simulink model "fft_wideband_real"  (R2012b)
settings: Solver=ode45  StartTime=0.0  StopTime=19999  RelTol=1e-3
undefined symbols (not defined in the file): fft_wideband_real_shift_schedule_user_data_out
libraries: xbsIndex_r4 x8703, xbsReplacements_r4 x36, xps_library x24, dspsigops x16, simulink_xsg_bridge x1
(part 5 of 51)

== system fft_wideband_real/fft_wideband_real/fft_direct/butterfly2_4 ==
  a : Inport
  b : Inport  Port=2
  w : Inport  Port=3
  sync : Inport  Port=4
  shift : Inport  Port=5
  AddSub0 : xbsIndex_r4/AddSub  mode=Addition  use_carryin=off  use_carryout=off  en=off  latency=2  precision=Full  arith_type=Unsigned  n_bits=16  bin_pt=14  quantization=Truncate  overflow=Wrap  dbl_ovrd=off  use_behavioral_HDL=on  hw_selection=Fabric  pipelined=off  block_type=addsub
  AddSub1 : xbsIndex_r4/AddSub  mode=Addition  use_carryin=off  use_carryout=off  en=off  latency=2  precision=Full  arith_type=Unsigned  n_bits=16  bin_pt=14  quantization=Truncate  overflow=Wrap  dbl_ovrd=off  use_behavioral_HDL=on  hw_selection=Fabric  pipelined=off  block_type=addsub
  AddSub2 : xbsIndex_r4/AddSub  mode=Subtraction  use_carryin=off  use_carryout=off  en=off  latency=2  precision=Full  arith_type=Unsigned  n_bits=16  bin_pt=14  quantization=Truncate  overflow=Wrap  dbl_ovrd=off  use_behavioral_HDL=on  hw_selection=Fabric  pipelined=off  block_type=addsub
  AddSub3 : xbsIndex_r4/AddSub  mode=Subtraction  use_carryin=off  use_carryout=off  en=off  latency=2  precision=Full  arith_type=Unsigned  n_bits=16  bin_pt=14  quantization=Truncate  overflow=Wrap  dbl_ovrd=off  use_behavioral_HDL=on  hw_selection=Fabric  pipelined=off  block_type=addsub
  Logical : xbsIndex_r4/Logical  logical_function=OR  inputs=4  en=off  latency=0  precision=Full  arith_type=Unsigned  n_bits=16  bin_pt=0  align_bp=on  dbl_ovrd=off  block_type=logical
  conv_of_1 : Subsystem
      settings: AttributesFormatString=[20,18]->[18,17]
  conv_of_2 : Subsystem
      settings: AttributesFormatString=[20,18]->[18,17]
  conv_of_3 : Subsystem
      settings: AttributesFormatString=[20,18]->[18,17]
  conv_of_4 : Subsystem
      settings: AttributesFormatString=[20,18]->[18,17]
  mux_{1..4} (4 alike) : xbsIndex_r4/Mux  inputs=2  en=off  latency=1  precision=Full  arith_type=Unsigned  n_bits=16  bin_pt=14  quantization=Truncate  overflow=Wrap  dbl_ovrd=off  block_type=mux
  ri_to_c01 : Subsystem
  ri_to_c23 : Subsystem
  scale_{1..4} (4 alike) : xbsIndex_r4/Scale  scale_factor=-1  dbl_ovrd=off  block_type=scale
  shift_del : xbsIndex_r4/Delay  rst=off  infoeditControl=Selection of Reset will increase slice count due to use of real FFs and instead of SRLs  en=off  latency=2  dbl_ovrd=off  reg_retiming=off  block_type=delay
  sync_delay : xbsIndex_r4/Delay  rst=off  infoeditControl=Selection of Reset will increase slice count due to use of real FFs and instead of SRLs  en=off  latency=4  dbl_ovrd=off  reg_retiming=on  block_type=delay
  twiddle : Subsystem
      settings: AttributesFormatString=twiddle_coeff_1
  a+bw : Outport
  a-bw : Outport  Port=2
  of : Outport  Port=3
  sync_out : Outport  Port=4
  wires:
  a/1 -> twiddle/1(a)
  b/1 -> twiddle/2(b)
  w/1 -> twiddle/3(w)
  sync/1 -> twiddle/4(sync)
  shift/1 -> shift_del/1
  scale_1/1 -> mux_1/3
  mux_1/1 -> conv_of_1/1(din)
  scale_2/1 -> mux_2/3
  mux_2/1 -> conv_of_2/1(din)
  scale_3/1 -> mux_3/3
  mux_3/1 -> conv_of_3/1(din)
  scale_4/1 -> mux_4/3
  mux_4/1 -> conv_of_4/1(din)
  conv_of_1/2(of) -> Logical/1
  conv_of_2/2(of) -> Logical/2
  conv_of_3/2(of) -> Logical/3
  conv_of_4/2(of) -> Logical/4
  Logical/1 -> of/1
  conv_of_1/1(dout) -> ri_to_c01/1(re)
  conv_of_2/1(dout) -> ri_to_c01/2(im)
  ri_to_c01/1(c) -> a+bw/1
  conv_of_3/1(dout) -> ri_to_c23/1(re)
  conv_of_4/1(dout) -> ri_to_c23/2(im)
  ri_to_c23/1(c) -> a-bw/1
  twiddle/5(sync_out) -> sync_delay/1  "twiddle_sync_out"
  sync_delay/1 -> sync_out/1
  AddSub3/1 -> scale_4/1, mux_4/2
  AddSub2/1 -> scale_3/1, mux_3/2
  AddSub1/1 -> scale_2/1, mux_2/2
  shift_del/1 -> mux_1/1, mux_2/1, mux_3/1, mux_4/1
  AddSub0/1 -> scale_1/1, mux_1/2
  twiddle/4(bw_im) -> AddSub1/2, AddSub3/2
  twiddle/2(a_im) -> AddSub1/1, AddSub3/1
  twiddle/3(bw_re) -> AddSub0/2, AddSub2/2
  twiddle/1(a_re) -> AddSub0/1, AddSub2/1

== system fft_wideband_real/fft_wideband_real/fft_direct/butterfly2_4_coef ==
  imag_const : xbsIndex_r4/Constant  const=-1  gui_display_data_type=Fixed-point  arith_type=Signed (2's comp)  n_bits=18  bin_pt=17  preci_type=Single  exp_width=8  frac_width=24  explicit_period=off  period=1  equ=P=C  opselect=C  inp2=PCIN>>17  opr=+  inp1=P  carry=CIN  dbl_ovrd=off  block_type=constant
  real_const : xbsIndex_r4/Constant  const=6.12323399573677e-17  gui_display_data_type=Fixed-point  arith_type=Signed (2's comp)  n_bits=18  bin_pt=17  preci_type=Single  exp_width=8  frac_width=24  explicit_period=off  period=1  equ=P=C  opselect=C  inp2=PCIN>>17  opr=+  inp1=P  carry=CIN  dbl_ovrd=off  block_type=constant
  ri_to_c : Subsystem
  out : Outport
  wires:
  real_const/1 -> ri_to_c/1(re)
  imag_const/1 -> ri_to_c/2(im)
  ri_to_c/1(c) -> out/1

== system fft_wideband_real/fft_wideband_real/fft_direct/butterfly2_5 ==
  a : Inport
  b : Inport  Port=2
  w : Inport  Port=3
  sync : Inport  Port=4
  shift : Inport  Port=5
  AddSub0 : xbsIndex_r4/AddSub  mode=Addition  use_carryin=off  use_carryout=off  en=off  latency=2  precision=Full  arith_type=Unsigned  n_bits=16  bin_pt=14  quantization=Truncate  overflow=Wrap  dbl_ovrd=off  use_behavioral_HDL=on  hw_selection=Fabric  pipelined=off  block_type=addsub
  AddSub1 : xbsIndex_r4/AddSub  mode=Addition  use_carryin=off  use_carryout=off  en=off  latency=2  precision=Full  arith_type=Unsigned  n_bits=16  bin_pt=14  quantization=Truncate  overflow=Wrap  dbl_ovrd=off  use_behavioral_HDL=on  hw_selection=Fabric  pipelined=off  block_type=addsub
  AddSub2 : xbsIndex_r4/AddSub  mode=Subtraction  use_carryin=off  use_carryout=off  en=off  latency=2  precision=Full  arith_type=Unsigned  n_bits=16  bin_pt=14  quantization=Truncate  overflow=Wrap  dbl_ovrd=off  use_behavioral_HDL=on  hw_selection=Fabric  pipelined=off  block_type=addsub
  AddSub3 : xbsIndex_r4/AddSub  mode=Subtraction  use_carryin=off  use_carryout=off  en=off  latency=2  precision=Full  arith_type=Unsigned  n_bits=16  bin_pt=14  quantization=Truncate  overflow=Wrap  dbl_ovrd=off  use_behavioral_HDL=on  hw_selection=Fabric  pipelined=off  block_type=addsub
  Logical : xbsIndex_r4/Logical  logical_function=OR  inputs=4  en=off  latency=0  precision=Full  arith_type=Unsigned  n_bits=16  bin_pt=0  align_bp=on  dbl_ovrd=off  block_type=logical
  conv_of_1 : Subsystem
      settings: AttributesFormatString=[20,18]->[18,17]
  conv_of_2 : Subsystem
      settings: AttributesFormatString=[20,18]->[18,17]
  conv_of_3 : Subsystem
      settings: AttributesFormatString=[20,18]->[18,17]
  conv_of_4 : Subsystem
      settings: AttributesFormatString=[20,18]->[18,17]
  mux_{1..4} (4 alike) : xbsIndex_r4/Mux  inputs=2  en=off  latency=1  precision=Full  arith_type=Unsigned  n_bits=16  bin_pt=14  quantization=Truncate  overflow=Wrap  dbl_ovrd=off  block_type=mux
  ri_to_c01 : Subsystem
  ri_to_c23 : Subsystem
  scale_{1..4} (4 alike) : xbsIndex_r4/Scale  scale_factor=-1  dbl_ovrd=off  block_type=scale
  shift_del : xbsIndex_r4/Delay  rst=off  infoeditControl=Selection of Reset will increase slice count due to use of real FFs and instead of SRLs  en=off  latency=2  dbl_ovrd=off  reg_retiming=off  block_type=delay
  sync_delay : xbsIndex_r4/Delay  rst=off  infoeditControl=Selection of Reset will increase slice count due to use of real FFs and instead of SRLs  en=off  latency=4  dbl_ovrd=off  reg_retiming=on  block_type=delay
  twiddle : Subsystem
      settings: AttributesFormatString=twiddle_coeff_1
  a+bw : Outport
  a-bw : Outport  Port=2
  of : Outport  Port=3
  sync_out : Outport  Port=4
  wires:
  a/1 -> twiddle/1(a)
  b/1 -> twiddle/2(b)
  w/1 -> twiddle/3(w)
  sync/1 -> twiddle/4(sync)
  shift/1 -> shift_del/1
  scale_1/1 -> mux_1/3
  mux_1/1 -> conv_of_1/1(din)
  scale_2/1 -> mux_2/3
  mux_2/1 -> conv_of_2/1(din)
  scale_3/1 -> mux_3/3
  mux_3/1 -> conv_of_3/1(din)
  scale_4/1 -> mux_4/3
  mux_4/1 -> conv_of_4/1(din)
  conv_of_1/2(of) -> Logical/1
  conv_of_2/2(of) -> Logical/2
  conv_of_3/2(of) -> Logical/3
  conv_of_4/2(of) -> Logical/4
  Logical/1 -> of/1
  conv_of_1/1(dout) -> ri_to_c01/1(re)
  conv_of_2/1(dout) -> ri_to_c01/2(im)
  ri_to_c01/1(c) -> a+bw/1
  conv_of_3/1(dout) -> ri_to_c23/1(re)
  conv_of_4/1(dout) -> ri_to_c23/2(im)
  ri_to_c23/1(c) -> a-bw/1
  twiddle/5(sync_out) -> sync_delay/1  "twiddle_sync_out"
  sync_delay/1 -> sync_out/1
  AddSub3/1 -> scale_4/1, mux_4/2
  AddSub2/1 -> scale_3/1, mux_3/2
  AddSub1/1 -> scale_2/1, mux_2/2
  shift_del/1 -> mux_1/1, mux_2/1, mux_3/1, mux_4/1
  AddSub0/1 -> scale_1/1, mux_1/2
  twiddle/4(bw_im) -> AddSub1/2, AddSub3/2
  twiddle/2(a_im) -> AddSub1/1, AddSub3/1
  twiddle/3(bw_re) -> AddSub0/2, AddSub2/2
  twiddle/1(a_re) -> AddSub0/1, AddSub2/1

== system fft_wideband_real/fft_wideband_real/fft_direct/butterfly2_5_coef ==
  imag_const : xbsIndex_r4/Constant  const=-1  gui_display_data_type=Fixed-point  arith_type=Signed (2's comp)  n_bits=18  bin_pt=17  preci_type=Single  exp_width=8  frac_width=24  explicit_period=off  period=1  equ=P=C  opselect=C  inp2=PCIN>>17  opr=+  inp1=P  carry=CIN  dbl_ovrd=off  block_type=constant
  real_const : xbsIndex_r4/Constant  const=6.12323399573677e-17  gui_display_data_type=Fixed-point  arith_type=Signed (2's comp)  n_bits=18  bin_pt=17  preci_type=Single  exp_width=8  frac_width=24  explicit_period=off  period=1  equ=P=C  opselect=C  inp2=PCIN>>17  opr=+  inp1=P  carry=CIN  dbl_ovrd=off  block_type=constant
  ri_to_c : Subsystem
  out : Outport
  wires:
  real_const/1 -> ri_to_c/1(re)
  imag_const/1 -> ri_to_c/2(im)
  ri_to_c/1(c) -> out/1

== system fft_wideband_real/fft_wideband_real/fft_direct/butterfly2_6 ==
  a : Inport
  b : Inport  Port=2
  w : Inport  Port=3
  sync : Inport  Port=4
  shift : Inport  Port=5
  AddSub0 : xbsIndex_r4/AddSub  mode=Addition  use_carryin=off  use_carryout=off  en=off  latency=2  precision=Full  arith_type=Unsigned  n_bits=16  bin_pt=14  quantization=Truncate  overflow=Wrap  dbl_ovrd=off  use_behavioral_HDL=on  hw_selection=Fabric  pipelined=off  block_type=addsub
  AddSub1 : xbsIndex_r4/AddSub  mode=Addition  use_carryin=off  use_carryout=off  en=off  latency=2  precision=Full  arith_type=Unsigned  n_bits=16  bin_pt=14  quantization=Truncate  overflow=Wrap  dbl_ovrd=off  use_behavioral_HDL=on  hw_selection=Fabric  pipelined=off  block_type=addsub
  AddSub2 : xbsIndex_r4/AddSub  mode=Subtraction  use_carryin=off  use_carryout=off  en=off  latency=2  precision=Full  arith_type=Unsigned  n_bits=16  bin_pt=14  quantization=Truncate  overflow=Wrap  dbl_ovrd=off  use_behavioral_HDL=on  hw_selection=Fabric  pipelined=off  block_type=addsub
  AddSub3 : xbsIndex_r4/AddSub  mode=Subtraction  use_carryin=off  use_carryout=off  en=off  latency=2  precision=Full  arith_type=Unsigned  n_bits=16  bin_pt=14  quantization=Truncate  overflow=Wrap  dbl_ovrd=off  use_behavioral_HDL=on  hw_selection=Fabric  pipelined=off  block_type=addsub
  Logical : xbsIndex_r4/Logical  logical_function=OR  inputs=4  en=off  latency=0  precision=Full  arith_type=Unsigned  n_bits=16  bin_pt=0  align_bp=on  dbl_ovrd=off  block_type=logical
  conv_of_1 : Subsystem
      settings: AttributesFormatString=[20,18]->[18,17]
  conv_of_2 : Subsystem
      settings: AttributesFormatString=[20,18]->[18,17]
  conv_of_3 : Subsystem
      settings: AttributesFormatString=[20,18]->[18,17]
  conv_of_4 : Subsystem
      settings: AttributesFormatString=[20,18]->[18,17]
  mux_{1..4} (4 alike) : xbsIndex_r4/Mux  inputs=2  en=off  latency=1  precision=Full  arith_type=Unsigned  n_bits=16  bin_pt=14  quantization=Truncate  overflow=Wrap  dbl_ovrd=off  block_type=mux
  ri_to_c01 : Subsystem
  ri_to_c23 : Subsystem
  scale_{1..4} (4 alike) : xbsIndex_r4/Scale  scale_factor=-1  dbl_ovrd=off  block_type=scale
  shift_del : xbsIndex_r4/Delay  rst=off  infoeditControl=Selection of Reset will increase slice count due to use of real FFs and instead of SRLs  en=off  latency=2  dbl_ovrd=off  reg_retiming=off  block_type=delay
  sync_delay : xbsIndex_r4/Delay  rst=off  infoeditControl=Selection of Reset will increase slice count due to use of real FFs and instead of SRLs  en=off  latency=4  dbl_ovrd=off  reg_retiming=on  block_type=delay
  twiddle : Subsystem
      settings: AttributesFormatString=twiddle_coeff_1
  a+bw : Outport
  a-bw : Outport  Port=2
  of : Outport  Port=3
  sync_out : Outport  Port=4
  wires:
  a/1 -> twiddle/1(a)
  b/1 -> twiddle/2(b)
  w/1 -> twiddle/3(w)
  sync/1 -> twiddle/4(sync)
  shift/1 -> shift_del/1
  scale_1/1 -> mux_1/3
  mux_1/1 -> conv_of_1/1(din)
  scale_2/1 -> mux_2/3
  mux_2/1 -> conv_of_2/1(din)
  scale_3/1 -> mux_3/3
  mux_3/1 -> conv_of_3/1(din)
  scale_4/1 -> mux_4/3
  mux_4/1 -> conv_of_4/1(din)
  conv_of_1/2(of) -> Logical/1
  conv_of_2/2(of) -> Logical/2
  conv_of_3/2(of) -> Logical/3
  conv_of_4/2(of) -> Logical/4
  Logical/1 -> of/1
  conv_of_1/1(dout) -> ri_to_c01/1(re)
  conv_of_2/1(dout) -> ri_to_c01/2(im)
  ri_to_c01/1(c) -> a+bw/1
  conv_of_3/1(dout) -> ri_to_c23/1(re)
  conv_of_4/1(dout) -> ri_to_c23/2(im)
  ri_to_c23/1(c) -> a-bw/1
  twiddle/5(sync_out) -> sync_delay/1  "twiddle_sync_out"
  sync_delay/1 -> sync_out/1
  AddSub3/1 -> scale_4/1, mux_4/2
  AddSub2/1 -> scale_3/1, mux_3/2
  AddSub1/1 -> scale_2/1, mux_2/2
  shift_del/1 -> mux_1/1, mux_2/1, mux_3/1, mux_4/1
  AddSub0/1 -> scale_1/1, mux_1/2
  twiddle/4(bw_im) -> AddSub1/2, AddSub3/2
  twiddle/2(a_im) -> AddSub1/1, AddSub3/1
  twiddle/3(bw_re) -> AddSub0/2, AddSub2/2
  twiddle/1(a_re) -> AddSub0/1, AddSub2/1

== system fft_wideband_real/fft_wideband_real/fft_direct/butterfly2_6_coef ==
  imag_const : xbsIndex_r4/Constant  const=-1  gui_display_data_type=Fixed-point  arith_type=Signed (2's comp)  n_bits=18  bin_pt=17  preci_type=Single  exp_width=8  frac_width=24  explicit_period=off  period=1  equ=P=C  opselect=C  inp2=PCIN>>17  opr=+  inp1=P  carry=CIN  dbl_ovrd=off  block_type=constant
  real_const : xbsIndex_r4/Constant  const=6.12323399573677e-17  gui_display_data_type=Fixed-point  arith_type=Signed (2's comp)  n_bits=18  bin_pt=17  preci_type=Single  exp_width=8  frac_width=24  explicit_period=off  period=1  equ=P=C  opselect=C  inp2=PCIN>>17  opr=+  inp1=P  carry=CIN  dbl_ovrd=off  block_type=constant
  ri_to_c : Subsystem
  out : Outport
  wires:
  real_const/1 -> ri_to_c/1(re)
  imag_const/1 -> ri_to_c/2(im)
  ri_to_c/1(c) -> out/1

== system fft_wideband_real/fft_wideband_real/fft_direct/butterfly2_7 ==
  a : Inport
  b : Inport  Port=2
  w : Inport  Port=3
  sync : Inport  Port=4
  shift : Inport  Port=5
  AddSub0 : xbsIndex_r4/AddSub  mode=Addition  use_carryin=off  use_carryout=off  en=off  latency=2  precision=Full  arith_type=Unsigned  n_bits=16  bin_pt=14  quantization=Truncate  overflow=Wrap  dbl_ovrd=off  use_behavioral_HDL=on  hw_selection=Fabric  pipelined=off  block_type=addsub
  AddSub1 : xbsIndex_r4/AddSub  mode=Addition  use_carryin=off  use_carryout=off  en=off  latency=2  precision=Full  arith_type=Unsigned  n_bits=16  bin_pt=14  quantization=Truncate  overflow=Wrap  dbl_ovrd=off  use_behavioral_HDL=on  hw_selection=Fabric  pipelined=off  block_type=addsub
  AddSub2 : xbsIndex_r4/AddSub  mode=Subtraction  use_carryin=off  use_carryout=off  en=off  latency=2  precision=Full  arith_type=Unsigned  n_bits=16  bin_pt=14  quantization=Truncate  overflow=Wrap  dbl_ovrd=off  use_behavioral_HDL=on  hw_selection=Fabric  pipelined=off  block_type=addsub
  AddSub3 : xbsIndex_r4/AddSub  mode=Subtraction  use_carryin=off  use_carryout=off  en=off  latency=2  precision=Full  arith_type=Unsigned  n_bits=16  bin_pt=14  quantization=Truncate  overflow=Wrap  dbl_ovrd=off  use_behavioral_HDL=on  hw_selection=Fabric  pipelined=off  block_type=addsub
  Logical : xbsIndex_r4/Logical  logical_function=OR  inputs=4  en=off  latency=0  precision=Full  arith_type=Unsigned  n_bits=16  bin_pt=0  align_bp=on  dbl_ovrd=off  block_type=logical
  conv_of_1 : Subsystem
      settings: AttributesFormatString=[20,18]->[18,17]
  conv_of_2 : Subsystem
      settings: AttributesFormatString=[20,18]->[18,17]
  conv_of_3 : Subsystem
      settings: AttributesFormatString=[20,18]->[18,17]
  conv_of_4 : Subsystem
      settings: AttributesFormatString=[20,18]->[18,17]
  mux_{1..4} (4 alike) : xbsIndex_r4/Mux  inputs=2  en=off  latency=1  precision=Full  arith_type=Unsigned  n_bits=16  bin_pt=14  quantization=Truncate  overflow=Wrap  dbl_ovrd=off  block_type=mux
  ri_to_c01 : Subsystem
  ri_to_c23 : Subsystem
  scale_{1..4} (4 alike) : xbsIndex_r4/Scale  scale_factor=-1  dbl_ovrd=off  block_type=scale
  shift_del : xbsIndex_r4/Delay  rst=off  infoeditControl=Selection of Reset will increase slice count due to use of real FFs and instead of SRLs  en=off  latency=2  dbl_ovrd=off  reg_retiming=off  block_type=delay
  sync_delay : xbsIndex_r4/Delay  rst=off  infoeditControl=Selection of Reset will increase slice count due to use of real FFs and instead of SRLs  en=off  latency=4  dbl_ovrd=off  reg_retiming=on  block_type=delay
  twiddle : Subsystem
      settings: AttributesFormatString=twiddle_coeff_1
  a+bw : Outport
  a-bw : Outport  Port=2
  of : Outport  Port=3
  sync_out : Outport  Port=4
  wires:
  a/1 -> twiddle/1(a)
  b/1 -> twiddle/2(b)
  w/1 -> twiddle/3(w)
  sync/1 -> twiddle/4(sync)
  shift/1 -> shift_del/1
  scale_1/1 -> mux_1/3
  mux_1/1 -> conv_of_1/1(din)
  scale_2/1 -> mux_2/3
  mux_2/1 -> conv_of_2/1(din)
  scale_3/1 -> mux_3/3
  mux_3/1 -> conv_of_3/1(din)
  scale_4/1 -> mux_4/3
  mux_4/1 -> conv_of_4/1(din)
  conv_of_1/2(of) -> Logical/1
  conv_of_2/2(of) -> Logical/2
  conv_of_3/2(of) -> Logical/3
  conv_of_4/2(of) -> Logical/4
  Logical/1 -> of/1
  conv_of_1/1(dout) -> ri_to_c01/1(re)
  conv_of_2/1(dout) -> ri_to_c01/2(im)
  ri_to_c01/1(c) -> a+bw/1
  conv_of_3/1(dout) -> ri_to_c23/1(re)
  conv_of_4/1(dout) -> ri_to_c23/2(im)
  ri_to_c23/1(c) -> a-bw/1
  twiddle/5(sync_out) -> sync_delay/1  "twiddle_sync_out"
  sync_delay/1 -> sync_out/1
  AddSub3/1 -> scale_4/1, mux_4/2
  AddSub2/1 -> scale_3/1, mux_3/2
  AddSub1/1 -> scale_2/1, mux_2/2
  shift_del/1 -> mux_1/1, mux_2/1, mux_3/1, mux_4/1
  AddSub0/1 -> scale_1/1, mux_1/2
  twiddle/4(bw_im) -> AddSub1/2, AddSub3/2
  twiddle/2(a_im) -> AddSub1/1, AddSub3/1
  twiddle/3(bw_re) -> AddSub0/2, AddSub2/2
  twiddle/1(a_re) -> AddSub0/1, AddSub2/1

== system fft_wideband_real/fft_wideband_real/fft_direct/butterfly2_7_coef ==
  imag_const : xbsIndex_r4/Constant  const=-1  gui_display_data_type=Fixed-point  arith_type=Signed (2's comp)  n_bits=18  bin_pt=17  preci_type=Single  exp_width=8  frac_width=24  explicit_period=off  period=1  equ=P=C  opselect=C  inp2=PCIN>>17  opr=+  inp1=P  carry=CIN  dbl_ovrd=off  block_type=constant
  real_const : xbsIndex_r4/Constant  const=6.12323399573677e-17  gui_display_data_type=Fixed-point  arith_type=Signed (2's comp)  n_bits=18  bin_pt=17  preci_type=Single  exp_width=8  frac_width=24  explicit_period=off  period=1  equ=P=C  opselect=C  inp2=PCIN>>17  opr=+  inp1=P  carry=CIN  dbl_ovrd=off  block_type=constant
  ri_to_c : Subsystem
  out : Outport
  wires:
  real_const/1 -> ri_to_c/1(re)
  imag_const/1 -> ri_to_c/2(im)
  ri_to_c/1(c) -> out/1

== system fft_wideband_real/fft_wideband_real/fft_direct/butterfly3_0 ==
  a : Inport
  b : Inport  Port=2
  w : Inport  Port=3
  sync : Inport  Port=4
  shift : Inport  Port=5
  AddSub0 : xbsIndex_r4/AddSub  mode=Addition  use_carryin=off  use_carryout=off  en=off  latency=2  precision=Full  arith_type=Unsigned  n_bits=16  bin_pt=14  quantization=Truncate  overflow=Wrap  dbl_ovrd=off  use_behavioral_HDL=on  hw_selection=Fabric  pipelined=off  block_type=addsub
  AddSub1 : xbsIndex_r4/AddSub  mode=Addition  use_carryin=off  use_carryout=off  en=off  latency=2  precision=Full  arith_type=Unsigned  n_bits=16  bin_pt=14  quantization=Truncate  overflow=Wrap  dbl_ovrd=off  use_behavioral_HDL=on  hw_selection=Fabric  pipelined=off  block_type=addsub
  AddSub2 : xbsIndex_r4/AddSub  mode=Subtraction  use_carryin=off  use_carryout=off  en=off  latency=2  precision=Full  arith_type=Unsigned  n_bits=16  bin_pt=14  quantization=Truncate  overflow=Wrap  dbl_ovrd=off  use_behavioral_HDL=on  hw_selection=Fabric  pipelined=off  block_type=addsub
  AddSub3 : xbsIndex_r4/AddSub  mode=Subtraction  use_carryin=off  use_carryout=off  en=off  latency=2  precision=Full  arith_type=Unsigned  n_bits=16  bin_pt=14  quantization=Truncate  overflow=Wrap  dbl_ovrd=off  use_behavioral_HDL=on  hw_selection=Fabric  pipelined=off  block_type=addsub
  Logical : xbsIndex_r4/Logical  logical_function=OR  inputs=4  en=off  latency=0  precision=Full  arith_type=Unsigned  n_bits=16  bin_pt=0  align_bp=on  dbl_ovrd=off  block_type=logical
  conv_of_1 : Subsystem
      settings: AttributesFormatString=[24,20]->[18,17]
  conv_of_2 : Subsystem
      settings: AttributesFormatString=[24,20]->[18,17]
  conv_of_3 : Subsystem
      settings: AttributesFormatString=[24,20]->[18,17]
  conv_of_4 : Subsystem
      settings: AttributesFormatString=[24,20]->[18,17]
  mux_{1..4} (4 alike) : xbsIndex_r4/Mux  inputs=2  en=off  latency=1  precision=Full  arith_type=Unsigned  n_bits=16  bin_pt=14  quantization=Truncate  overflow=Wrap  dbl_ovrd=off  block_type=mux
  ri_to_c01 : Subsystem
  ri_to_c23 : Subsystem
  scale_{1..4} (4 alike) : xbsIndex_r4/Scale  scale_factor=-1  dbl_ovrd=off  block_type=scale
  shift_del : xbsIndex_r4/Delay  rst=off  infoeditControl=Selection of Reset will increase slice count due to use of real FFs and instead of SRLs  en=off  latency=2  dbl_ovrd=off  reg_retiming=off  block_type=delay
  sync_delay : xbsIndex_r4/Delay  rst=off  infoeditControl=Selection of Reset will increase slice count due to use of real FFs and instead of SRLs  en=off  latency=4  dbl_ovrd=off  reg_retiming=on  block_type=delay
  twiddle : Subsystem
      settings: AttributesFormatString=|
      | data=(18,17)
      | coeffs=(18,16)
      | Virtex5
      | (Round  (unbiased: +/- Inf),Saturate)
      | twiddle_general_4mult
  a+bw : Outport
  a-bw : Outport  Port=2
  of : Outport  Port=3
  sync_out : Outport  Port=4
  wires:
  a/1 -> twiddle/1(a)
  b/1 -> twiddle/2(b)
  w/1 -> twiddle/3(w)
  sync/1 -> twiddle/4(sync)
  shift/1 -> shift_del/1
  scale_1/1 -> mux_1/3
  mux_1/1 -> conv_of_1/1(din)
  scale_2/1 -> mux_2/3
  mux_2/1 -> conv_of_2/1(din)
  scale_3/1 -> mux_3/3
  mux_3/1 -> conv_of_3/1(din)
  scale_4/1 -> mux_4/3
  mux_4/1 -> conv_of_4/1(din)
  conv_of_1/2(of) -> Logical/1
  conv_of_2/2(of) -> Logical/2
  conv_of_3/2(of) -> Logical/3
  conv_of_4/2(of) -> Logical/4
  Logical/1 -> of/1
  conv_of_1/1(dout) -> ri_to_c01/1(re)
  conv_of_2/1(dout) -> ri_to_c01/2(im)
  ri_to_c01/1(c) -> a+bw/1
  conv_of_3/1(dout) -> ri_to_c23/1(re)
  conv_of_4/1(dout) -> ri_to_c23/2(im)
  ri_to_c23/1(c) -> a-bw/1
  twiddle/5(sync_out) -> sync_delay/1  "twiddle_sync_out"
  sync_delay/1 -> sync_out/1
  AddSub3/1 -> scale_4/1, mux_4/2
  AddSub2/1 -> scale_3/1, mux_3/2
  AddSub1/1 -> scale_2/1, mux_2/2
  shift_del/1 -> mux_1/1, mux_2/1, mux_3/1, mux_4/1
  AddSub0/1 -> scale_1/1, mux_1/2
  twiddle/4(bw_im) -> AddSub1/2, AddSub3/2
  twiddle/2(a_im) -> AddSub1/1, AddSub3/1
  twiddle/3(bw_re) -> AddSub0/2, AddSub2/2
  twiddle/1(a_re) -> AddSub0/1, AddSub2/1

== system fft_wideband_real/fft_wideband_real/fft_direct/butterfly3_0_coef ==
  imag_const : xbsIndex_r4/Constant  const=0  gui_display_data_type=Fixed-point  arith_type=Signed (2's comp)  n_bits=18  bin_pt=17  preci_type=Single  exp_width=8  frac_width=24  explicit_period=off  period=1  equ=P=C  opselect=C  inp2=PCIN>>17  opr=+  inp1=P  carry=CIN  dbl_ovrd=off  block_type=constant
  real_const : xbsIndex_r4/Constant  const=1  gui_display_data_type=Fixed-point  arith_type=Signed (2's comp)  n_bits=18  bin_pt=17  preci_type=Single  exp_width=8  frac_width=24  explicit_period=off  period=1  equ=P=C  opselect=C  inp2=PCIN>>17  opr=+  inp1=P  carry=CIN  dbl_ovrd=off  block_type=constant
  ri_to_c : Subsystem
  out : Outport
  wires:
  real_const/1 -> ri_to_c/1(re)
  imag_const/1 -> ri_to_c/2(im)
  ri_to_c/1(c) -> out/1

== system fft_wideband_real/fft_wideband_real/fft_direct/butterfly3_1 ==
  a : Inport
  b : Inport  Port=2
  w : Inport  Port=3
  sync : Inport  Port=4
  shift : Inport  Port=5
  AddSub0 : xbsIndex_r4/AddSub  mode=Addition  use_carryin=off  use_carryout=off  en=off  latency=2  precision=Full  arith_type=Unsigned  n_bits=16  bin_pt=14  quantization=Truncate  overflow=Wrap  dbl_ovrd=off  use_behavioral_HDL=on  hw_selection=Fabric  pipelined=off  block_type=addsub
  AddSub1 : xbsIndex_r4/AddSub  mode=Addition  use_carryin=off  use_carryout=off  en=off  latency=2  precision=Full  arith_type=Unsigned  n_bits=16  bin_pt=14  quantization=Truncate  overflow=Wrap  dbl_ovrd=off  use_behavioral_HDL=on  hw_selection=Fabric  pipelined=off  block_type=addsub
  AddSub2 : xbsIndex_r4/AddSub  mode=Subtraction  use_carryin=off  use_carryout=off  en=off  latency=2  precision=Full  arith_type=Unsigned  n_bits=16  bin_pt=14  quantization=Truncate  overflow=Wrap  dbl_ovrd=off  use_behavioral_HDL=on  hw_selection=Fabric  pipelined=off  block_type=addsub
  AddSub3 : xbsIndex_r4/AddSub  mode=Subtraction  use_carryin=off  use_carryout=off  en=off  latency=2  precision=Full  arith_type=Unsigned  n_bits=16  bin_pt=14  quantization=Truncate  overflow=Wrap  dbl_ovrd=off  use_behavioral_HDL=on  hw_selection=Fabric  pipelined=off  block_type=addsub
  Logical : xbsIndex_r4/Logical  logical_function=OR  inputs=4  en=off  latency=0  precision=Full  arith_type=Unsigned  n_bits=16  bin_pt=0  align_bp=on  dbl_ovrd=off  block_type=logical
  conv_of_1 : Subsystem
      settings: AttributesFormatString=[24,20]->[18,17]
  conv_of_2 : Subsystem
      settings: AttributesFormatString=[24,20]->[18,17]
  conv_of_3 : Subsystem
      settings: AttributesFormatString=[24,20]->[18,17]
  conv_of_4 : Subsystem
      settings: AttributesFormatString=[24,20]->[18,17]
  mux_{1..4} (4 alike) : xbsIndex_r4/Mux  inputs=2  en=off  latency=1  precision=Full  arith_type=Unsigned  n_bits=16  bin_pt=14  quantization=Truncate  overflow=Wrap  dbl_ovrd=off  block_type=mux
  ri_to_c01 : Subsystem
  ri_to_c23 : Subsystem
  scale_{1..4} (4 alike) : xbsIndex_r4/Scale  scale_factor=-1  dbl_ovrd=off  block_type=scale
  shift_del : xbsIndex_r4/Delay  rst=off  infoeditControl=Selection of Reset will increase slice count due to use of real FFs and instead of SRLs  en=off  latency=2  dbl_ovrd=off  reg_retiming=off  block_type=delay
  sync_delay : xbsIndex_r4/Delay  rst=off  infoeditControl=Selection of Reset will increase slice count due to use of real FFs and instead of SRLs  en=off  latency=4  dbl_ovrd=off  reg_retiming=on  block_type=delay
  twiddle : Subsystem
      settings: AttributesFormatString=|
      | data=(18,17)
      | coeffs=(18,16)
      | Virtex5
      | (Round  (unbiased: +/- Inf),Saturate)
      | twiddle_general_4mult
  a+bw : Outport
  a-bw : Outport  Port=2
  of : Outport  Port=3
  sync_out : Outport  Port=4
  wires:
  a/1 -> twiddle/1(a)
  b/1 -> twiddle/2(b)
  w/1 -> twiddle/3(w)
  sync/1 -> twiddle/4(sync)
  shift/1 -> shift_del/1
  scale_1/1 -> mux_1/3
  mux_1/1 -> conv_of_1/1(din)
  scale_2/1 -> mux_2/3
  mux_2/1 -> conv_of_2/1(din)
  scale_3/1 -> mux_3/3
  mux_3/1 -> conv_of_3/1(din)
  scale_4/1 -> mux_4/3
  mux_4/1 -> conv_of_4/1(din)
  conv_of_1/2(of) -> Logical/1
  conv_of_2/2(of) -> Logical/2
  conv_of_3/2(of) -> Logical/3
  conv_of_4/2(of) -> Logical/4
  Logical/1 -> of/1
  conv_of_1/1(dout) -> ri_to_c01/1(re)
  conv_of_2/1(dout) -> ri_to_c01/2(im)
  ri_to_c01/1(c) -> a+bw/1
  conv_of_3/1(dout) -> ri_to_c23/1(re)
  conv_of_4/1(dout) -> ri_to_c23/2(im)
  ri_to_c23/1(c) -> a-bw/1
  twiddle/5(sync_out) -> sync_delay/1  "twiddle_sync_out"
  sync_delay/1 -> sync_out/1
  AddSub3/1 -> scale_4/1, mux_4/2
  AddSub2/1 -> scale_3/1, mux_3/2
  AddSub1/1 -> scale_2/1, mux_2/2
  shift_del/1 -> mux_1/1, mux_2/1, mux_3/1, mux_4/1
  AddSub0/1 -> scale_1/1, mux_1/2
  twiddle/4(bw_im) -> AddSub1/2, AddSub3/2
  twiddle/2(a_im) -> AddSub1/1, AddSub3/1
  twiddle/3(bw_re) -> AddSub0/2, AddSub2/2
  twiddle/1(a_re) -> AddSub0/1, AddSub2/1

== system fft_wideband_real/fft_wideband_real/fft_direct/butterfly3_1_coef ==
  imag_const : xbsIndex_r4/Constant  const=0  gui_display_data_type=Fixed-point  arith_type=Signed (2's comp)  n_bits=18  bin_pt=17  preci_type=Single  exp_width=8  frac_width=24  explicit_period=off  period=1  equ=P=C  opselect=C  inp2=PCIN>>17  opr=+  inp1=P  carry=CIN  dbl_ovrd=off  block_type=constant
  real_const : xbsIndex_r4/Constant  const=1  gui_display_data_type=Fixed-point  arith_type=Signed (2's comp)  n_bits=18  bin_pt=17  preci_type=Single  exp_width=8  frac_width=24  explicit_period=off  period=1  equ=P=C  opselect=C  inp2=PCIN>>17  opr=+  inp1=P  carry=CIN  dbl_ovrd=off  block_type=constant
  ri_to_c : Subsystem
  out : Outport
  wires:
  real_const/1 -> ri_to_c/1(re)
  imag_const/1 -> ri_to_c/2(im)
  ri_to_c/1(c) -> out/1

== system fft_wideband_real/fft_wideband_real/fft_direct/butterfly3_2 ==
  a : Inport
  b : Inport  Port=2
  w : Inport  Port=3
  sync : Inport  Port=4
  shift : Inport  Port=5
  AddSub0 : xbsIndex_r4/AddSub  mode=Addition  use_carryin=off  use_carryout=off  en=off  latency=2  precision=Full  arith_type=Unsigned  n_bits=16  bin_pt=14  quantization=Truncate  overflow=Wrap  dbl_ovrd=off  use_behavioral_HDL=on  hw_selection=Fabric  pipelined=off  block_type=addsub
  AddSub1 : xbsIndex_r4/AddSub  mode=Addition  use_carryin=off  use_carryout=off  en=off  latency=2  precision=Full  arith_type=Unsigned  n_bits=16  bin_pt=14  quantization=Truncate  overflow=Wrap  dbl_ovrd=off  use_behavioral_HDL=on  hw_selection=Fabric  pipelined=off  block_type=addsub
  AddSub2 : xbsIndex_r4/AddSub  mode=Subtraction  use_carryin=off  use_carryout=off  en=off  latency=2  precision=Full  arith_type=Unsigned  n_bits=16  bin_pt=14  quantization=Truncate  overflow=Wrap  dbl_ovrd=off  use_behavioral_HDL=on  hw_selection=Fabric  pipelined=off  block_type=addsub
  AddSub3 : xbsIndex_r4/AddSub  mode=Subtraction  use_carryin=off  use_carryout=off  en=off  latency=2  precision=Full  arith_type=Unsigned  n_bits=16  bin_pt=14  quantization=Truncate  overflow=Wrap  dbl_ovrd=off  use_behavioral_HDL=on  hw_selection=Fabric  pipelined=off  block_type=addsub
  Logical : xbsIndex_r4/Logical  logical_function=OR  inputs=4  en=off  latency=0  precision=Full  arith_type=Unsigned  n_bits=16  bin_pt=0  align_bp=on  dbl_ovrd=off  block_type=logical
  conv_of_1 : Subsystem
      settings: AttributesFormatString=[24,20]->[18,17]
  conv_of_2 : Subsystem
      settings: AttributesFormatString=[24,20]->[18,17]
  conv_of_3 : Subsystem
      settings: AttributesFormatString=[24,20]->[18,17]
  conv_of_4 : Subsystem
      settings: AttributesFormatString=[24,20]->[18,17]
  mux_{1..4} (4 alike) : xbsIndex_r4/Mux  inputs=2  en=off  latency=1  precision=Full  arith_type=Unsigned  n_bits=16  bin_pt=14  quantization=Truncate  overflow=Wrap  dbl_ovrd=off  block_type=mux
  ri_to_c01 : Subsystem
  ri_to_c23 : Subsystem
  scale_{1..4} (4 alike) : xbsIndex_r4/Scale  scale_factor=-1  dbl_ovrd=off  block_type=scale
  shift_del : xbsIndex_r4/Delay  rst=off  infoeditControl=Selection of Reset will increase slice count due to use of real FFs and instead of SRLs  en=off  latency=2  dbl_ovrd=off  reg_retiming=off  block_type=delay
  sync_delay : xbsIndex_r4/Delay  rst=off  infoeditControl=Selection of Reset will increase slice count due to use of real FFs and instead of SRLs  en=off  latency=4  dbl_ovrd=off  reg_retiming=on  block_type=delay
  twiddle : Subsystem
      settings: AttributesFormatString=|
      | data=(18,17)
      | coeffs=(18,16)
      | Virtex5
      | (Round  (unbiased: +/- Inf),Saturate)
      | twiddle_general_4mult
  a+bw : Outport
  a-bw : Outport  Port=2
  of : Outport  Port=3
  sync_out : Outport  Port=4
  wires:
  a/1 -> twiddle/1(a)
  b/1 -> twiddle/2(b)
  w/1 -> twiddle/3(w)
  sync/1 -> twiddle/4(sync)
  shift/1 -> shift_del/1
  scale_1/1 -> mux_1/3
  mux_1/1 -> conv_of_1/1(din)
  scale_2/1 -> mux_2/3
  mux_2/1 -> conv_of_2/1(din)
  scale_3/1 -> mux_3/3
  mux_3/1 -> conv_of_3/1(din)
  scale_4/1 -> mux_4/3
  mux_4/1 -> conv_of_4/1(din)
  conv_of_1/2(of) -> Logical/1
  conv_of_2/2(of) -> Logical/2
  conv_of_3/2(of) -> Logical/3
  conv_of_4/2(of) -> Logical/4
  Logical/1 -> of/1
  conv_of_1/1(dout) -> ri_to_c01/1(re)
  conv_of_2/1(dout) -> ri_to_c01/2(im)
  ri_to_c01/1(c) -> a+bw/1
  conv_of_3/1(dout) -> ri_to_c23/1(re)
  conv_of_4/1(dout) -> ri_to_c23/2(im)
  ri_to_c23/1(c) -> a-bw/1
  twiddle/5(sync_out) -> sync_delay/1  "twiddle_sync_out"
  sync_delay/1 -> sync_out/1
  AddSub3/1 -> scale_4/1, mux_4/2
  AddSub2/1 -> scale_3/1, mux_3/2
  AddSub1/1 -> scale_2/1, mux_2/2
  shift_del/1 -> mux_1/1, mux_2/1, mux_3/1, mux_4/1
  AddSub0/1 -> scale_1/1, mux_1/2
  twiddle/4(bw_im) -> AddSub1/2, AddSub3/2
  twiddle/2(a_im) -> AddSub1/1, AddSub3/1
  twiddle/3(bw_re) -> AddSub0/2, AddSub2/2
  twiddle/1(a_re) -> AddSub0/1, AddSub2/1

== system fft_wideband_real/fft_wideband_real/fft_direct/butterfly3_2_coef ==
  imag_const : xbsIndex_r4/Constant  const=-1  gui_display_data_type=Fixed-point  arith_type=Signed (2's comp)  n_bits=18  bin_pt=17  preci_type=Single  exp_width=8  frac_width=24  explicit_period=off  period=1  equ=P=C  opselect=C  inp2=PCIN>>17  opr=+  inp1=P  carry=CIN  dbl_ovrd=off  block_type=constant
  real_const : xbsIndex_r4/Constant  const=6.12323399573677e-17  gui_display_data_type=Fixed-point  arith_type=Signed (2's comp)  n_bits=18  bin_pt=17  preci_type=Single  exp_width=8  frac_width=24  explicit_period=off  period=1  equ=P=C  opselect=C  inp2=PCIN>>17  opr=+  inp1=P  carry=CIN  dbl_ovrd=off  block_type=constant
  ri_to_c : Subsystem
  out : Outport
  wires:
  real_const/1 -> ri_to_c/1(re)
  imag_const/1 -> ri_to_c/2(im)
  ri_to_c/1(c) -> out/1

== system fft_wideband_real/fft_wideband_real/fft_direct/butterfly3_3 ==
  a : Inport
  b : Inport  Port=2
  w : Inport  Port=3
  sync : Inport  Port=4
  shift : Inport  Port=5
  AddSub0 : xbsIndex_r4/AddSub  mode=Addition  use_carryin=off  use_carryout=off  en=off  latency=2  precision=Full  arith_type=Unsigned  n_bits=16  bin_pt=14  quantization=Truncate  overflow=Wrap  dbl_ovrd=off  use_behavioral_HDL=on  hw_selection=Fabric  pipelined=off  block_type=addsub
  AddSub1 : xbsIndex_r4/AddSub  mode=Addition  use_carryin=off  use_carryout=off  en=off  latency=2  precision=Full  arith_type=Unsigned  n_bits=16  bin_pt=14  quantization=Truncate  overflow=Wrap  dbl_ovrd=off  use_behavioral_HDL=on  hw_selection=Fabric  pipelined=off  block_type=addsub
  AddSub2 : xbsIndex_r4/AddSub  mode=Subtraction  use_carryin=off  use_carryout=off  en=off  latency=2  precision=Full  arith_type=Unsigned  n_bits=16  bin_pt=14  quantization=Truncate  overflow=Wrap  dbl_ovrd=off  use_behavioral_HDL=on  hw_selection=Fabric  pipelined=off  block_type=addsub
  AddSub3 : xbsIndex_r4/AddSub  mode=Subtraction  use_carryin=off  use_carryout=off  en=off  latency=2  precision=Full  arith_type=Unsigned  n_bits=16  bin_pt=14  quantization=Truncate  overflow=Wrap  dbl_ovrd=off  use_behavioral_HDL=on  hw_selection=Fabric  pipelined=off  block_type=addsub
  Logical : xbsIndex_r4/Logical  logical_function=OR  inputs=4  en=off  latency=0  precision=Full  arith_type=Unsigned  n_bits=16  bin_pt=0  align_bp=on  dbl_ovrd=off  block_type=logical
  conv_of_1 : Subsystem
      settings: AttributesFormatString=[24,20]->[18,17]
  conv_of_2 : Subsystem
      settings: AttributesFormatString=[24,20]->[18,17]
  conv_of_3 : Subsystem
      settings: AttributesFormatString=[24,20]->[18,17]
  conv_of_4 : Subsystem
      settings: AttributesFormatString=[24,20]->[18,17]
  mux_{1..4} (4 alike) : xbsIndex_r4/Mux  inputs=2  en=off  latency=1  precision=Full  arith_type=Unsigned  n_bits=16  bin_pt=14  quantization=Truncate  overflow=Wrap  dbl_ovrd=off  block_type=mux
  ri_to_c01 : Subsystem
  ri_to_c23 : Subsystem
  scale_{1..4} (4 alike) : xbsIndex_r4/Scale  scale_factor=-1  dbl_ovrd=off  block_type=scale
  shift_del : xbsIndex_r4/Delay  rst=off  infoeditControl=Selection of Reset will increase slice count due to use of real FFs and instead of SRLs  en=off  latency=2  dbl_ovrd=off  reg_retiming=off  block_type=delay
  sync_delay : xbsIndex_r4/Delay  rst=off  infoeditControl=Selection of Reset will increase slice count due to use of real FFs and instead of SRLs  en=off  latency=4  dbl_ovrd=off  reg_retiming=on  block_type=delay
  twiddle : Subsystem
      settings: AttributesFormatString=|
      | data=(18,17)
      | coeffs=(18,16)
      | Virtex5
      | (Round  (unbiased: +/- Inf),Saturate)
      | twiddle_general_4mult
  a+bw : Outport
  a-bw : Outport  Port=2
  of : Outport  Port=3
  sync_out : Outport  Port=4
  wires:
  a/1 -> twiddle/1(a)
  b/1 -> twiddle/2(b)
  w/1 -> twiddle/3(w)
  sync/1 -> twiddle/4(sync)
  shift/1 -> shift_del/1
  scale_1/1 -> mux_1/3
  mux_1/1 -> conv_of_1/1(din)
  scale_2/1 -> mux_2/3
  mux_2/1 -> conv_of_2/1(din)
  scale_3/1 -> mux_3/3
  mux_3/1 -> conv_of_3/1(din)
  scale_4/1 -> mux_4/3
  mux_4/1 -> conv_of_4/1(din)
  conv_of_1/2(of) -> Logical/1
  conv_of_2/2(of) -> Logical/2
  conv_of_3/2(of) -> Logical/3
  conv_of_4/2(of) -> Logical/4
  Logical/1 -> of/1
  conv_of_1/1(dout) -> ri_to_c01/1(re)
  conv_of_2/1(dout) -> ri_to_c01/2(im)
  ri_to_c01/1(c) -> a+bw/1
  conv_of_3/1(dout) -> ri_to_c23/1(re)
  conv_of_4/1(dout) -> ri_to_c23/2(im)
  ri_to_c23/1(c) -> a-bw/1
  twiddle/5(sync_out) -> sync_delay/1  "twiddle_sync_out"
  sync_delay/1 -> sync_out/1
  AddSub3/1 -> scale_4/1, mux_4/2
  AddSub2/1 -> scale_3/1, mux_3/2
  AddSub1/1 -> scale_2/1, mux_2/2
  shift_del/1 -> mux_1/1, mux_2/1, mux_3/1, mux_4/1
  AddSub0/1 -> scale_1/1, mux_1/2
  twiddle/4(bw_im) -> AddSub1/2, AddSub3/2
  twiddle/2(a_im) -> AddSub1/1, AddSub3/1
  twiddle/3(bw_re) -> AddSub0/2, AddSub2/2
  twiddle/1(a_re) -> AddSub0/1, AddSub2/1

== system fft_wideband_real/fft_wideband_real/fft_direct/butterfly3_3_coef ==
  imag_const : xbsIndex_r4/Constant  const=-1  gui_display_data_type=Fixed-point  arith_type=Signed (2's comp)  n_bits=18  bin_pt=17  preci_type=Single  exp_width=8  frac_width=24  explicit_period=off  period=1  equ=P=C  opselect=C  inp2=PCIN>>17  opr=+  inp1=P  carry=CIN  dbl_ovrd=off  block_type=constant
  real_const : xbsIndex_r4/Constant  const=6.12323399573677e-17  gui_display_data_type=Fixed-point  arith_type=Signed (2's comp)  n_bits=18  bin_pt=17  preci_type=Single  exp_width=8  frac_width=24  explicit_period=off  period=1  equ=P=C  opselect=C  inp2=PCIN>>17  opr=+  inp1=P  carry=CIN  dbl_ovrd=off  block_type=constant
  ri_to_c : Subsystem
  out : Outport
  wires:
  real_const/1 -> ri_to_c/1(re)
  imag_const/1 -> ri_to_c/2(im)
  ri_to_c/1(c) -> out/1

== system fft_wideband_real/fft_wideband_real/fft_direct/butterfly3_4 ==
  a : Inport
  b : Inport  Port=2
  w : Inport  Port=3
  sync : Inport  Port=4
  shift : Inport  Port=5
  AddSub0 : xbsIndex_r4/AddSub  mode=Addition  use_carryin=off  use_carryout=off  en=off  latency=2  precision=Full  arith_type=Unsigned  n_bits=16  bin_pt=14  quantization=Truncate  overflow=Wrap  dbl_ovrd=off  use_behavioral_HDL=on  hw_selection=Fabric  pipelined=off  block_type=addsub
  AddSub1 : xbsIndex_r4/AddSub  mode=Addition  use_carryin=off  use_carryout=off  en=off  latency=2  precision=Full  arith_type=Unsigned  n_bits=16  bin_pt=14  quantization=Truncate  overflow=Wrap  dbl_ovrd=off  use_behavioral_HDL=on  hw_selection=Fabric  pipelined=off  block_type=addsub
  AddSub2 : xbsIndex_r4/AddSub  mode=Subtraction  use_carryin=off  use_carryout=off  en=off  latency=2  precision=Full  arith_type=Unsigned  n_bits=16  bin_pt=14  quantization=Truncate  overflow=Wrap  dbl_ovrd=off  use_behavioral_HDL=on  hw_selection=Fabric  pipelined=off  block_type=addsub
  AddSub3 : xbsIndex_r4/AddSub  mode=Subtraction  use_carryin=off  use_carryout=off  en=off  latency=2  precision=Full  arith_type=Unsigned  n_bits=16  bin_pt=14  quantization=Truncate  overflow=Wrap  dbl_ovrd=off  use_behavioral_HDL=on  hw_selection=Fabric  pipelined=off  block_type=addsub
  Logical : xbsIndex_r4/Logical  logical_function=OR  inputs=4  en=off  latency=0  precision=Full  arith_type=Unsigned  n_bits=16  bin_pt=0  align_bp=on  dbl_ovrd=off  block_type=logical
  conv_of_1 : Subsystem
      settings: AttributesFormatString=[24,20]->[18,17]
  conv_of_2 : Subsystem
      settings: AttributesFormatString=[24,20]->[18,17]
  conv_of_3 : Subsystem
      settings: AttributesFormatString=[24,20]->[18,17]
  conv_of_4 : Subsystem
      settings: AttributesFormatString=[24,20]->[18,17]
  mux_{1..4} (4 alike) : xbsIndex_r4/Mux  inputs=2  en=off  latency=1  precision=Full  arith_type=Unsigned  n_bits=16  bin_pt=14  quantization=Truncate  overflow=Wrap  dbl_ovrd=off  block_type=mux
  ri_to_c01 : Subsystem
  ri_to_c23 : Subsystem
  scale_{1..4} (4 alike) : xbsIndex_r4/Scale  scale_factor=-1  dbl_ovrd=off  block_type=scale
  shift_del : xbsIndex_r4/Delay  rst=off  infoeditControl=Selection of Reset will increase slice count due to use of real FFs and instead of SRLs  en=off  latency=2  dbl_ovrd=off  reg_retiming=off  block_type=delay
  sync_delay : xbsIndex_r4/Delay  rst=off  infoeditControl=Selection of Reset will increase slice count due to use of real FFs and instead of SRLs  en=off  latency=4  dbl_ovrd=off  reg_retiming=on  block_type=delay
  twiddle : Subsystem
      settings: AttributesFormatString=|
      | data=(18,17)
      | coeffs=(18,16)
      | Virtex5
      | (Round  (unbiased: +/- Inf),Saturate)
      | twiddle_general_4mult
  a+bw : Outport
  a-bw : Outport  Port=2
  of : Outport  Port=3
  sync_out : Outport  Port=4
  wires:
  a/1 -> twiddle/1(a)
  b/1 -> twiddle/2(b)
  w/1 -> twiddle/3(w)
  sync/1 -> twiddle/4(sync)
  shift/1 -> shift_del/1
  scale_1/1 -> mux_1/3
  mux_1/1 -> conv_of_1/1(din)
  scale_2/1 -> mux_2/3
  mux_2/1 -> conv_of_2/1(din)
  scale_3/1 -> mux_3/3
  mux_3/1 -> conv_of_3/1(din)
  scale_4/1 -> mux_4/3
  mux_4/1 -> conv_of_4/1(din)
  conv_of_1/2(of) -> Logical/1
  conv_of_2/2(of) -> Logical/2
  conv_of_3/2(of) -> Logical/3
  conv_of_4/2(of) -> Logical/4
  Logical/1 -> of/1
  conv_of_1/1(dout) -> ri_to_c01/1(re)
  conv_of_2/1(dout) -> ri_to_c01/2(im)
  ri_to_c01/1(c) -> a+bw/1
  conv_of_3/1(dout) -> ri_to_c23/1(re)
  conv_of_4/1(dout) -> ri_to_c23/2(im)
  ri_to_c23/1(c) -> a-bw/1
  twiddle/5(sync_out) -> sync_delay/1  "twiddle_sync_out"
  sync_delay/1 -> sync_out/1
  AddSub3/1 -> scale_4/1, mux_4/2
  AddSub2/1 -> scale_3/1, mux_3/2
  AddSub1/1 -> scale_2/1, mux_2/2
  shift_del/1 -> mux_1/1, mux_2/1, mux_3/1, mux_4/1
  AddSub0/1 -> scale_1/1, mux_1/2
  twiddle/4(bw_im) -> AddSub1/2, AddSub3/2
  twiddle/2(a_im) -> AddSub1/1, AddSub3/1
  twiddle/3(bw_re) -> AddSub0/2, AddSub2/2
  twiddle/1(a_re) -> AddSub0/1, AddSub2/1

== system fft_wideband_real/fft_wideband_real/fft_direct/butterfly3_4_coef ==
  imag_const : xbsIndex_r4/Constant  const=-0.707106781186547  gui_display_data_type=Fixed-point  arith_type=Signed (2's comp)  n_bits=18  bin_pt=17  preci_type=Single  exp_width=8  frac_width=24  explicit_period=off  period=1  equ=P=C  opselect=C  inp2=PCIN>>17  opr=+  inp1=P  carry=CIN  dbl_ovrd=off  block_type=constant
  real_const : xbsIndex_r4/Constant  const=0.707106781186548  gui_display_data_type=Fixed-point  arith_type=Signed (2's comp)  n_bits=18  bin_pt=17  preci_type=Single  exp_width=8  frac_width=24  explicit_period=off  period=1  equ=P=C  opselect=C  inp2=PCIN>>17  opr=+  inp1=P  carry=CIN  dbl_ovrd=off  block_type=constant
  ri_to_c : Subsystem
  out : Outport
  wires:
  real_const/1 -> ri_to_c/1(re)
  imag_const/1 -> ri_to_c/2(im)
  ri_to_c/1(c) -> out/1

== system fft_wideband_real/fft_wideband_real/fft_direct/butterfly3_5 ==
  a : Inport
  b : Inport  Port=2
  w : Inport  Port=3
  sync : Inport  Port=4
  shift : Inport  Port=5
  AddSub0 : xbsIndex_r4/AddSub  mode=Addition  use_carryin=off  use_carryout=off  en=off  latency=2  precision=Full  arith_type=Unsigned  n_bits=16  bin_pt=14  quantization=Truncate  overflow=Wrap  dbl_ovrd=off  use_behavioral_HDL=on  hw_selection=Fabric  pipelined=off  block_type=addsub
  AddSub1 : xbsIndex_r4/AddSub  mode=Addition  use_carryin=off  use_carryout=off  en=off  latency=2  precision=Full  arith_type=Unsigned  n_bits=16  bin_pt=14  quantization=Truncate  overflow=Wrap  dbl_ovrd=off  use_behavioral_HDL=on  hw_selection=Fabric  pipelined=off  block_type=addsub
  AddSub2 : xbsIndex_r4/AddSub  mode=Subtraction  use_carryin=off  use_carryout=off  en=off  latency=2  precision=Full  arith_type=Unsigned  n_bits=16  bin_pt=14  quantization=Truncate  overflow=Wrap  dbl_ovrd=off  use_behavioral_HDL=on  hw_selection=Fabric  pipelined=off  block_type=addsub
  AddSub3 : xbsIndex_r4/AddSub  mode=Subtraction  use_carryin=off  use_carryout=off  en=off  latency=2  precision=Full  arith_type=Unsigned  n_bits=16  bin_pt=14  quantization=Truncate  overflow=Wrap  dbl_ovrd=off  use_behavioral_HDL=on  hw_selection=Fabric  pipelined=off  block_type=addsub
  Logical : xbsIndex_r4/Logical  logical_function=OR  inputs=4  en=off  latency=0  precision=Full  arith_type=Unsigned  n_bits=16  bin_pt=0  align_bp=on  dbl_ovrd=off  block_type=logical
  conv_of_1 : Subsystem
      settings: AttributesFormatString=[24,20]->[18,17]
  conv_of_2 : Subsystem
      settings: AttributesFormatString=[24,20]->[18,17]
  conv_of_3 : Subsystem
      settings: AttributesFormatString=[24,20]->[18,17]
  conv_of_4 : Subsystem
      settings: AttributesFormatString=[24,20]->[18,17]
  mux_{1..4} (4 alike) : xbsIndex_r4/Mux  inputs=2  en=off  latency=1  precision=Full  arith_type=Unsigned  n_bits=16  bin_pt=14  quantization=Truncate  overflow=Wrap  dbl_ovrd=off  block_type=mux
  ri_to_c01 : Subsystem
  ri_to_c23 : Subsystem
  scale_{1..4} (4 alike) : xbsIndex_r4/Scale  scale_factor=-1  dbl_ovrd=off  block_type=scale
  shift_del : xbsIndex_r4/Delay  rst=off  infoeditControl=Selection of Reset will increase slice count due to use of real FFs and instead of SRLs  en=off  latency=2  dbl_ovrd=off  reg_retiming=off  block_type=delay
  sync_delay : xbsIndex_r4/Delay  rst=off  infoeditControl=Selection of Reset will increase slice count due to use of real FFs and instead of SRLs  en=off  latency=4  dbl_ovrd=off  reg_retiming=on  block_type=delay
  twiddle : Subsystem
      settings: AttributesFormatString=|
      | data=(18,17)
      | coeffs=(18,16)
      | Virtex5
      | (Round  (unbiased: +/- Inf),Saturate)
      | twiddle_general_4mult
  a+bw : Outport
  a-bw : Outport  Port=2
  of : Outport  Port=3
  sync_out : Outport  Port=4
  wires:
  a/1 -> twiddle/1(a)
  b/1 -> twiddle/2(b)
  w/1 -> twiddle/3(w)
  sync/1 -> twiddle/4(sync)
  shift/1 -> shift_del/1
  scale_1/1 -> mux_1/3
  mux_1/1 -> conv_of_1/1(din)
  scale_2/1 -> mux_2/3
  mux_2/1 -> conv_of_2/1(din)
  scale_3/1 -> mux_3/3
  mux_3/1 -> conv_of_3/1(din)
  scale_4/1 -> mux_4/3
  mux_4/1 -> conv_of_4/1(din)
  conv_of_1/2(of) -> Logical/1
  conv_of_2/2(of) -> Logical/2
  conv_of_3/2(of) -> Logical/3
  conv_of_4/2(of) -> Logical/4
  Logical/1 -> of/1
  conv_of_1/1(dout) -> ri_to_c01/1(re)
  conv_of_2/1(dout) -> ri_to_c01/2(im)
  ri_to_c01/1(c) -> a+bw/1
  conv_of_3/1(dout) -> ri_to_c23/1(re)
  conv_of_4/1(dout) -> ri_to_c23/2(im)
  ri_to_c23/1(c) -> a-bw/1
  twiddle/5(sync_out) -> sync_delay/1  "twiddle_sync_out"
  sync_delay/1 -> sync_out/1
  AddSub3/1 -> scale_4/1, mux_4/2
  AddSub2/1 -> scale_3/1, mux_3/2
  AddSub1/1 -> scale_2/1, mux_2/2
  shift_del/1 -> mux_1/1, mux_2/1, mux_3/1, mux_4/1
  AddSub0/1 -> scale_1/1, mux_1/2
  twiddle/4(bw_im) -> AddSub1/2, AddSub3/2
  twiddle/2(a_im) -> AddSub1/1, AddSub3/1
  twiddle/3(bw_re) -> AddSub0/2, AddSub2/2
  twiddle/1(a_re) -> AddSub0/1, AddSub2/1

== system fft_wideband_real/fft_wideband_real/fft_direct/butterfly3_5_coef ==
  imag_const : xbsIndex_r4/Constant  const=-0.707106781186547  gui_display_data_type=Fixed-point  arith_type=Signed (2's comp)  n_bits=18  bin_pt=17  preci_type=Single  exp_width=8  frac_width=24  explicit_period=off  period=1  equ=P=C  opselect=C  inp2=PCIN>>17  opr=+  inp1=P  carry=CIN  dbl_ovrd=off  block_type=constant
  real_const : xbsIndex_r4/Constant  const=0.707106781186548  gui_display_data_type=Fixed-point  arith_type=Signed (2's comp)  n_bits=18  bin_pt=17  preci_type=Single  exp_width=8  frac_width=24  explicit_period=off  period=1  equ=P=C  opselect=C  inp2=PCIN>>17  opr=+  inp1=P  carry=CIN  dbl_ovrd=off  block_type=constant
  ri_to_c : Subsystem
  out : Outport
  wires:
  real_const/1 -> ri_to_c/1(re)
  imag_const/1 -> ri_to_c/2(im)
  ri_to_c/1(c) -> out/1
